simulink model "sys2"  (Simulink 7.7)
settings: Solver=ode45  StartTime=0.0  StopTime=5  RelTol=1e-3
values from neighbouring files (symbols this model uses):
  disturbance = 0    [case1.m]    (also in case2.m)
  input = null_in    [case1.m]    (also in case2.m)
  noise = .1    (= 0.1)    [case1.m]    (also in case2.m)
  p_den = conv([1 1 0], [0.1 1])    [main.m]
  p_num = 100    [main.m]
  q0 = [1 (N/k_d) 0]    [case2.m]
  q1 = [k_p (k_i + N * k_p/k_d) (N * k_i/k_d)]    [case2.m]
  q2 = [(N+k_p) (k_i+N*k_p/k_d) (N*k_i/k_d)]    [case2.m]
libraries: simulink x1
settings Model: Creator=Edward  LastModifiedBy=Edward

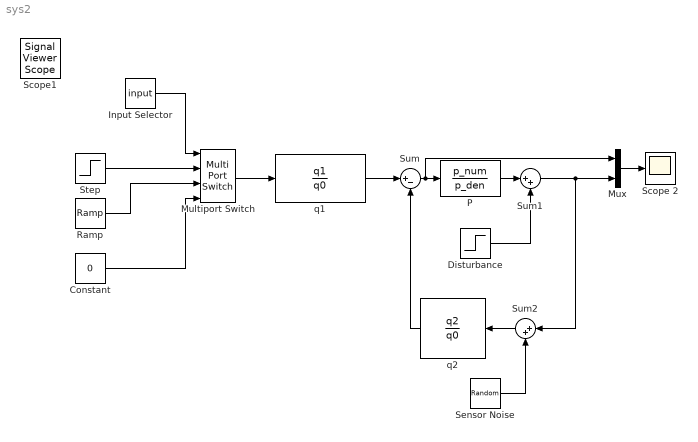
== system sys2 ==
  Constant : Constant  Value=0
  Disturbance : Step  After=disturbance  SampleTime=0
  Input Selector : Constant  Value=input
  Multiport Switch : MultiPortSwitch  zeroidx=off
  Mux : Mux  Inputs=2
  P : TransferFcn  Numerator=p_num  Denominator=p_den
  Ramp : simulink/Sources/Ramp  SystemSampleTime=-1  slope=1  start=0  X0=0
  Scope 2 : Scope
  Sensor Noise : RandomNumber  Variance=noise  SampleTime=0.01
  Step : Step  Time=0  SampleTime=0
  Sum : Sum  Inputs=|+-
  Sum1 : Sum  Inputs=|++
  Sum2 : Sum  Inputs=|++
  q1 : TransferFcn  Numerator=q1  Denominator=q0
  q2 : TransferFcn  Numerator=q2  Denominator=q0
  Scope1 : SignalViewerScope  IOType=viewer  RefreshTime=0.035000
  wires:
  Sum/1 -> P/1, Mux/1
  q1/1 -> Sum/1
  q2/1 -> Sum/2
  P/1 -> Sum1/1
  Sum2/1 -> q2/1
  Sum1/1 -> Sum2/1, Mux/2
  Sensor Noise/1 -> Sum2/2
  Disturbance/1 -> Sum1/2
  Step/1 -> Multiport Switch/2
  Ramp/1 -> Multiport Switch/3
  Input Selector/1 -> Multiport Switch/1
  Constant/1 -> Multiport Switch/4
  Multiport Switch/1 -> q1/1
  Mux/1 -> Scope 2/1
